simulink library "ddc_library"  (Simulink 6.2)
values from neighbouring files (symbols this model uses):
  num_fir_col = length(lpfir_coeff)/num_inputs    [ddc_mask.m]
libraries: xbsIndex_r3 x31, ddc_library x27, ddc_lo_lib x8
settings Model: LastModifiedBy=hchen05

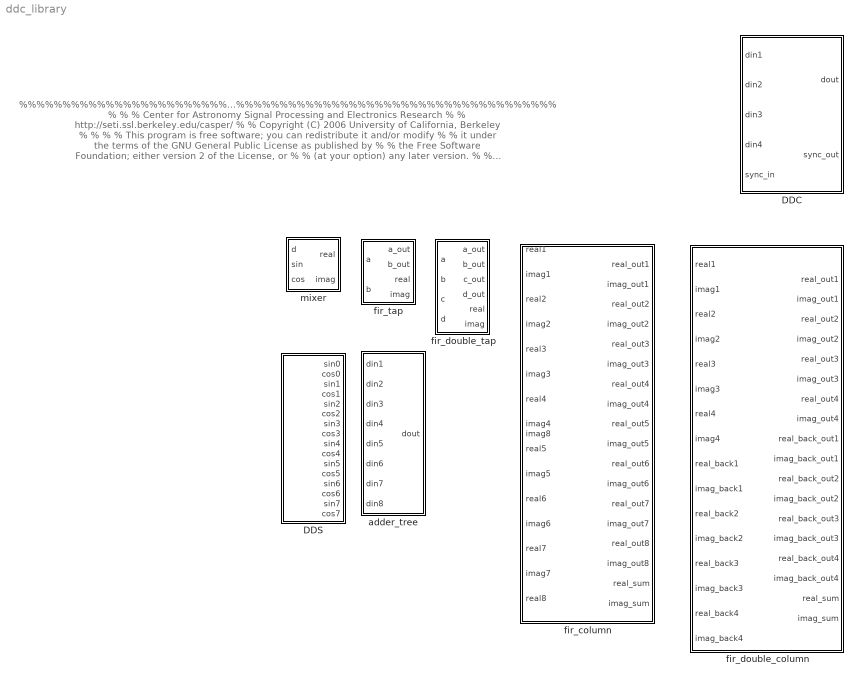
== system ddc_library ==
  note: %%%%%%%%%%%%%%%%%%%%%%%%%%%%%%%%%%%%%%%%%%%%%%%%%%%%%%%%%%%%%%%%%%%%%%%%%%%%%%%
      | %                                                                             %
      | %   Center for Astronomy Signal Processing and Electronics Research           %
      | %   http://seti.ssl.berkeley.edu/casper/                                      %
      | %   Copyright (C) 2006 University of California, Berkeley                     %
      | %                                                                             %
      | %   This program is free software; you can redistribute it and/or modify      %
      | %   it under the terms of the GNU General Public License as published by      %
      | %   the Free Software Foundation; either version 2 of the License, or         %
      | %   (at your option) any later version.                                       %
      | %                                                                             %
      | %   This program is distributed in the hope that it will be useful,           %
      | %   but WITHOUT ANY WARRANTY; without even the implied warranty of            %
      | %   MERCHANTABILITY or FITNESS FOR A PARTICULAR PURPOSE.  See the             %
      | %   GNU General Public License for more details.                              %
      | %                                                                             %
      | %   You should have received a copy of the GNU General Public License along   %
      | %   with this program; if not, write to the Free Software Foundation, Inc.,   %
      | %   51 Franklin Street, Fifth Floor, Boston, MA 02110-1301 USA.               %
      | %                                                                             %
      | %%%%%%%%%%%%%%%%%%%%%%%%%%%%%%%%%%%%%%%%%%%%%%%%%%%%%%%%%%%%%%%%%%%%%%%%%%%%%%%
  DDC : Subsystem  mask(DDC){freq_div=16, lo_freq=3, num_inputs=4, lo_bitwidth=18, lpfir_coeff=[1,zeros(1,15)], BitWidthOut=8, quantization=Round  (unbiased: +/- Inf), add_latency=2, mult_latency=3}
      mask prompts: freq_div "Frequency Divisions (M)"; lo_freq "LO Frequency (1/M*2pi)"; num_inputs "Inputs"; lo_bitwidth "LO BitWidth"; lpfir_coeff "FIR coefficients"; BitWidthOut "Bit Width Out"; quantization "Quantization Behavior"; add_latency "Add Latency"; mult_latency "Mult Latency"
      mask help: Decimating digital downconverter with parameterized LO and LPF coefficients.
      mask init:
      | ddc_mask;
      mask Help: eval('xlWeb([getenv(''MLIB_ROOT''), ''\astro_library\doc\ddc_usage.html''])')
      mask StyleString: edit,edit,edit,edit,edit,edit,popup(Truncate|Round  (unbiased: +/- Inf)|Round  (unbiased: Even Values)),edit,edit
  DDS : Subsystem  mask{freq_div=8, freq=2, num_lo=8, BitWidth=18, latency=2}
      mask prompts: freq_div "Frequency divisions (M)"; freq "Frequency (1/M*2pi)"; num_lo "Parallel LOs (N)"
      mask init:
      | dds_mask;
  adder_tree : Subsystem  mask{num_inputs=8, latency=2}
      mask prompts: num_inputs "Inputs"; latency "Latency per adder tree"
      mask init:
      | adder_tree_mask;
  fir_column : Subsystem  mask(fir_column){num_inputs=8, coeff=rand(128), mult_latency=2, add_latency=1}
      mask prompts: num_inputs "Inputs"; coeff "Coefficients"; mult_latency "Mult Latency"; add_latency "Add latency"
      mask init:
      | fir_column_mask;
  fir_double_column : Subsystem  mask(fir_double_column){num_inputs=4, coeff=rand(8), mult_latency=3, add_latency=2}
      mask prompts: num_inputs "Inputs"; coeff "Coefficients"; mult_latency "Mult Latency"; add_latency "Add latency"
      mask init:
      | fir_double_column_mask;
  fir_double_tap : Subsystem  mask(fir_double_tap){factor=0.073384, mult_latency=3, add_latency=2}
      mask prompts: mult_latency "Mult latency"; add_latency "Add latency"
  fir_tap : Subsystem  mask(fir_tap){factor=1, latency=3}
      mask prompts: latency "mult_latency"
  mixer : Subsystem  mask{BitWidth=18, latency=2}

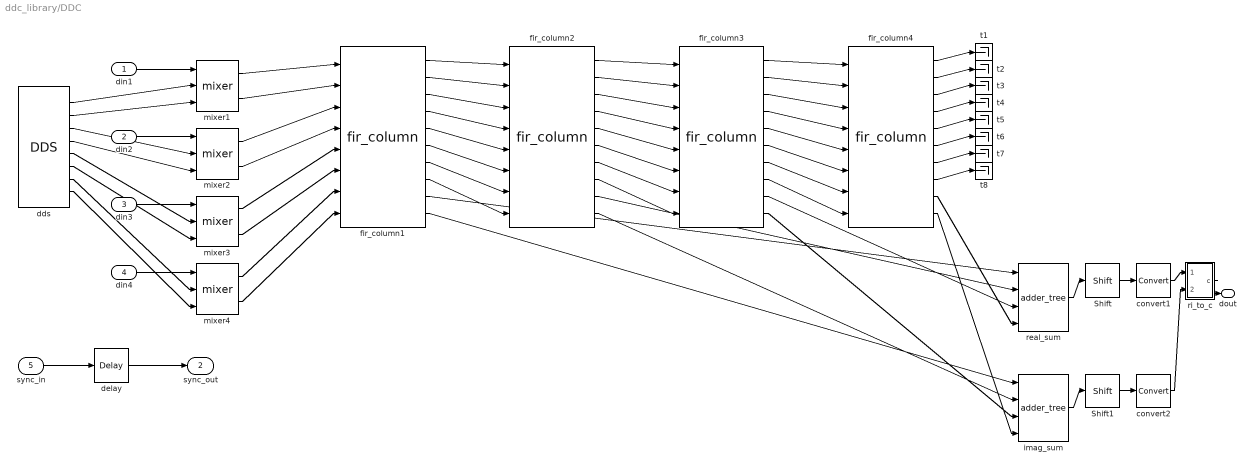
== system ddc_library/DDC ==
  din1 : Inport  Port=1  LatchInput=off
  din2 : Inport  Port=2  LatchInput=off
  din3 : Inport  Port=3  LatchInput=off
  din4 : Inport  Port=4  LatchInput=off
  sync_in : Inport  Port=5  LatchInput=off
  Shift : xbsIndex_r3/Shift  shift_dir=Left  shift_bits=1  precision=Full  arith_type="Signed  (2's comp)"  n_bits=8  bin_pt=2  quantization=Truncate  overflow=Wrap  latency=0  explicit_period=off  period=1  en=off  dbl_ovrd=off  show_param=off
      settings: xl_area=[0, 0, 0, 0, 0, 0, 0]
  Shift1 : xbsIndex_r3/Shift  shift_dir=Left  shift_bits=1  precision=Full  arith_type="Signed  (2's comp)"  n_bits=8  bin_pt=2  quantization=Truncate  overflow=Wrap  latency=0  explicit_period=off  period=1  en=off  dbl_ovrd=off  show_param=off
      settings: xl_area=[0, 0, 0, 0, 0, 0, 0]
  convert1 : xbsIndex_r3/Convert  arith_type="Signed  (2's comp)"  n_bits=BitWidthOut  bin_pt=BitWidthOut - 1  quantization="Round  (unbiased: +/- Inf)"  overflow=Saturate  latency=add_latency  explicit_period=on  period=1  dbl_ovrd=off  show_param=on  inserted_by_tool=off  pipeline=on
      settings: xl_area=[0, 0, 0, 0, 0, 0, 0]
  convert2 : xbsIndex_r3/Convert  arith_type="Signed  (2's comp)"  n_bits=BitWidthOut  bin_pt=BitWidthOut - 1  quantization="Round  (unbiased: +/- Inf)"  overflow=Saturate  latency=add_latency  explicit_period=on  period=1  dbl_ovrd=off  show_param=on  inserted_by_tool=off  pipeline=on
      settings: xl_area=[0, 0, 0, 0, 0, 0, 0]
  dds : ddc_library/DDS  freq_div=freq_div  freq=lo_freq  num_lo=num_inputs  BitWidth=lo_bitwidth  latency=2
      link override ddc_lo0/ddc_lo_const/const1: equ=P=C
  delay : xbsIndex_r3/Delay  latency=mult_latency*2+ceil(log2(num_inputs))*add_latency+ceil(log2(num_fir_col))*add_latency+add_latency  reg_retiming=off  explicit_period=off  period=1  en=off  accept_only_valid=off  init_zero=on  dbl_ovrd=off  show_param=off
      settings: xl_area=[0, 0, 0, 0, 0, 0, 0]
  fir_column1 : ddc_library/fir_column  num_inputs=num_inputs  coeff=lpfir_coeff(4:-1:1)  mult_latency=mult_latency  add_latency=1
  fir_column2 : ddc_library/fir_column  num_inputs=num_inputs  coeff=lpfir_coeff(8:-1:5)  mult_latency=mult_latency  add_latency=1
  fir_column3 : ddc_library/fir_column  num_inputs=num_inputs  coeff=lpfir_coeff(12:-1:9)  mult_latency=mult_latency  add_latency=1
  fir_column4 : ddc_library/fir_column  num_inputs=num_inputs  coeff=lpfir_coeff(16:-1:13)  mult_latency=mult_latency  add_latency=1
  imag_sum : ddc_library/adder_tree  num_inputs=4  latency=2
  mixer{1..4} (4 alike) : ddc_library/mixer  BitWidth=lo_bitwidth  latency=mult_latency
  real_sum : ddc_library/adder_tree  num_inputs=4  latency=2
  ri_to_c : Subsystem
  t{1..8} (8 alike) : Terminator
  dout : Outport
  sync_out : Outport  Port=2
  wires:
  real_sum/1 -> Shift/1
  imag_sum/1 -> Shift1/1
  Shift/1 -> convert1/1
  Shift1/1 -> convert2/1
  convert1/1 -> ri_to_c/1(re)
  convert2/1 -> ri_to_c/2(im)
  ri_to_c/1(c) -> dout/1
  sync_in/1 -> delay/1
  delay/1 -> sync_out/1
  din1/1 -> mixer1/1
  dds/1 -> mixer1/2
  dds/2 -> mixer1/3
  din2/1 -> mixer2/1
  dds/3 -> mixer2/2
  dds/4 -> mixer2/3
  din3/1 -> mixer3/1
  dds/5 -> mixer3/2
  dds/6 -> mixer3/3
  din4/1 -> mixer4/1
  dds/7 -> mixer4/2
  dds/8 -> mixer4/3
  mixer1/1 -> fir_column1/1
  mixer1/2 -> fir_column1/2
  mixer2/1 -> fir_column1/3
  mixer2/2 -> fir_column1/4
  mixer3/1 -> fir_column1/5
  mixer3/2 -> fir_column1/6
  mixer4/1 -> fir_column1/7
  mixer4/2 -> fir_column1/8
  fir_column1/9 -> real_sum/1
  fir_column1/10 -> imag_sum/1
  fir_column1/1 -> fir_column2/1
  fir_column1/2 -> fir_column2/2
  fir_column1/3 -> fir_column2/3
  fir_column1/4 -> fir_column2/4
  fir_column1/5 -> fir_column2/5
  fir_column1/6 -> fir_column2/6
  fir_column1/7 -> fir_column2/7
  fir_column1/8 -> fir_column2/8
  fir_column2/9 -> real_sum/2
  fir_column2/10 -> imag_sum/2
  fir_column2/1 -> fir_column3/1
  fir_column2/2 -> fir_column3/2
  fir_column2/3 -> fir_column3/3
  fir_column2/4 -> fir_column3/4
  fir_column2/5 -> fir_column3/5
  fir_column2/6 -> fir_column3/6
  fir_column2/7 -> fir_column3/7
  fir_column2/8 -> fir_column3/8
  fir_column3/9 -> real_sum/3
  fir_column3/10 -> imag_sum/3
  fir_column3/1 -> fir_column4/1
  fir_column3/2 -> fir_column4/2
  fir_column3/3 -> fir_column4/3
  fir_column3/4 -> fir_column4/4
  fir_column3/5 -> fir_column4/5
  fir_column3/6 -> fir_column4/6
  fir_column3/7 -> fir_column4/7
  fir_column3/8 -> fir_column4/8
  fir_column4/9 -> real_sum/4
  fir_column4/10 -> imag_sum/4
  fir_column4/1 -> t1/1
  fir_column4/2 -> t2/1
  fir_column4/3 -> t3/1
  fir_column4/4 -> t4/1
  fir_column4/5 -> t5/1
  fir_column4/6 -> t6/1
  fir_column4/7 -> t7/1
  fir_column4/8 -> t8/1

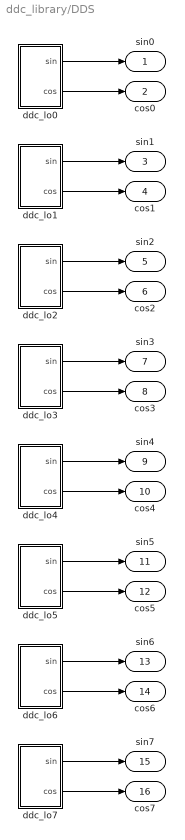
== system ddc_library/DDS ==
  ddc_lo0 : Subsystem  BlockChoice=ddc_lo_const
      link override ddc_lo_const: BitWidth=BitWidth  Phase=0
      link override ddc_lo_const/const1: equ=P=C
      link override ddc_lo_osc: BitWidth=BitWidth  counter_step=counter_step  counter_start=0  counter_width=counter_width  latency=latency
      settings: AttributesFormatString=%<BlockChoice>  TemplateBlock=ddc_lo_lib/ddc_lo  MemberBlocks=ddc_lo_const,ddc_lo_osc
  ddc_lo1 : Subsystem  BlockChoice=ddc_lo_const
      link override ddc_lo_const: BitWidth=BitWidth  Phase=1.5708
      link override ddc_lo_osc: BitWidth=BitWidth  counter_step=counter_step  counter_start=1  counter_width=counter_width  latency=latency
      settings: AttributesFormatString=%<BlockChoice>  TemplateBlock=ddc_lo_lib/ddc_lo  MemberBlocks=ddc_lo_const,ddc_lo_osc
  ddc_lo2 : Subsystem  BlockChoice=ddc_lo_const
      link override ddc_lo_const: BitWidth=BitWidth  Phase=3.1416
      link override ddc_lo_osc: BitWidth=BitWidth  counter_step=counter_step  counter_start=2  counter_width=counter_width  latency=latency
      settings: AttributesFormatString=%<BlockChoice>  TemplateBlock=ddc_lo_lib/ddc_lo  MemberBlocks=ddc_lo_const,ddc_lo_osc
  ddc_lo3 : Subsystem  BlockChoice=ddc_lo_const
      link override ddc_lo_const: BitWidth=BitWidth  Phase=4.7124
      link override ddc_lo_osc: BitWidth=BitWidth  counter_step=counter_step  counter_start=3  counter_width=counter_width  latency=latency
      settings: AttributesFormatString=%<BlockChoice>  TemplateBlock=ddc_lo_lib/ddc_lo  MemberBlocks=ddc_lo_const,ddc_lo_osc
  ddc_lo4 : Subsystem  BlockChoice=ddc_lo_const
      link override ddc_lo_const: BitWidth=BitWidth  Phase=6.2832
      settings: AttributesFormatString=%<BlockChoice>  TemplateBlock=ddc_lo_lib/ddc_lo  MemberBlocks=ddc_lo_const,ddc_lo_osc
  ddc_lo5 : Subsystem  BlockChoice=ddc_lo_const
      link override ddc_lo_const: BitWidth=BitWidth  Phase=7.854
      settings: AttributesFormatString=%<BlockChoice>  TemplateBlock=ddc_lo_lib/ddc_lo  MemberBlocks=ddc_lo_const,ddc_lo_osc
  ddc_lo6 : Subsystem  BlockChoice=ddc_lo_const
      link override ddc_lo_const: BitWidth=BitWidth  Phase=9.4248
      settings: AttributesFormatString=%<BlockChoice>  TemplateBlock=ddc_lo_lib/ddc_lo  MemberBlocks=ddc_lo_const,ddc_lo_osc
  ddc_lo7 : Subsystem  BlockChoice=ddc_lo_const
      link override ddc_lo_const: BitWidth=BitWidth  Phase=10.9956
      settings: AttributesFormatString=%<BlockChoice>  TemplateBlock=ddc_lo_lib/ddc_lo  MemberBlocks=ddc_lo_const,ddc_lo_osc
  sin0 : Outport
  cos0 : Outport  Port=2
  sin1 : Outport  Port=3
  cos1 : Outport  Port=4
  sin2 : Outport  Port=5
  cos2 : Outport  Port=6
  sin3 : Outport  Port=7
  cos3 : Outport  Port=8
  sin4 : Outport  Port=9
  cos4 : Outport  Port=10
  sin5 : Outport  Port=11
  cos5 : Outport  Port=12
  sin6 : Outport  Port=13
  cos6 : Outport  Port=14
  sin7 : Outport  Port=15
  cos7 : Outport  Port=16
  wires:
  ddc_lo0/1(sin) -> sin0/1
  ddc_lo0/2(cos) -> cos0/1
  ddc_lo1/1(sin) -> sin1/1
  ddc_lo1/2(cos) -> cos1/1
  ddc_lo2/1(sin) -> sin2/1
  ddc_lo2/2(cos) -> cos2/1
  ddc_lo3/1(sin) -> sin3/1
  ddc_lo3/2(cos) -> cos3/1
  ddc_lo4/1(sin) -> sin4/1
  ddc_lo4/2(cos) -> cos4/1
  ddc_lo5/1(sin) -> sin5/1
  ddc_lo5/2(cos) -> cos5/1
  ddc_lo6/1(sin) -> sin6/1
  ddc_lo6/2(cos) -> cos6/1
  ddc_lo7/1(sin) -> sin7/1
  ddc_lo7/2(cos) -> cos7/1

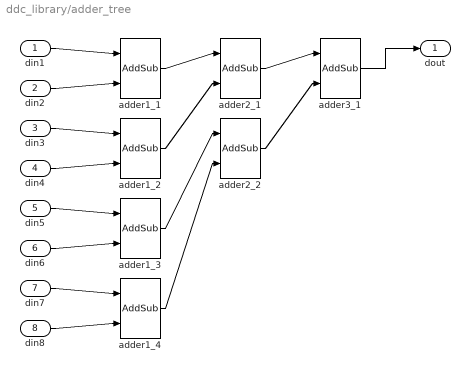
== system ddc_library/adder_tree ==
  din1 : Inport  Port=1  LatchInput=off
  din2 : Inport  Port=2  LatchInput=off
  din3 : Inport  Port=3  LatchInput=off
  din4 : Inport  Port=4  LatchInput=off
  din5 : Inport  Port=5  LatchInput=off
  din6 : Inport  Port=6  LatchInput=off
  din7 : Inport  Port=7  LatchInput=off
  din8 : Inport  Port=8  LatchInput=off
  adder1_{1..4} (4 alike) : xbsIndex_r3/AddSub  mode=Addition  precision=Full  arith_type=Unsigned  n_bits=8  bin_pt=2  quantization=Truncate  overflow=Wrap  latency=latency  explicit_period=off  period=1  use_carryin=off  use_carryout=off  en=off  dbl_ovrd=off  show_param=off  use_core=on  pipeline=on  use_rpm=on  gen_core=off
      settings: xl_area=[0, 0, 0, 0, 0, 0, 0]
  adder2_1 : xbsIndex_r3/AddSub  mode=Addition  precision=Full  arith_type=Unsigned  n_bits=8  bin_pt=2  quantization=Truncate  overflow=Wrap  latency=latency  explicit_period=off  period=1  use_carryin=off  use_carryout=off  en=off  dbl_ovrd=off  show_param=off  use_core=on  pipeline=on  use_rpm=on  gen_core=off
      settings: xl_area=[0, 0, 0, 0, 0, 0, 0]
  adder2_2 : xbsIndex_r3/AddSub  mode=Addition  precision=Full  arith_type=Unsigned  n_bits=8  bin_pt=2  quantization=Truncate  overflow=Wrap  latency=latency  explicit_period=off  period=1  use_carryin=off  use_carryout=off  en=off  dbl_ovrd=off  show_param=off  use_core=on  pipeline=on  use_rpm=on  gen_core=off
      settings: xl_area=[0, 0, 0, 0, 0, 0, 0]
  adder3_1 : xbsIndex_r3/AddSub  mode=Addition  precision=Full  arith_type=Unsigned  n_bits=8  bin_pt=2  quantization=Truncate  overflow=Wrap  latency=latency  explicit_period=off  period=1  use_carryin=off  use_carryout=off  en=off  dbl_ovrd=off  show_param=off  use_core=on  pipeline=on  use_rpm=on  gen_core=off
      settings: xl_area=[0, 0, 0, 0, 0, 0, 0]
  dout : Outport
  wires:
  din1/1 -> adder1_1/1
  din2/1 -> adder1_1/2
  din3/1 -> adder1_2/1
  din4/1 -> adder1_2/2
  din5/1 -> adder1_3/1
  din6/1 -> adder1_3/2
  din7/1 -> adder1_4/1
  din8/1 -> adder1_4/2
  adder1_1/1 -> adder2_1/1
  adder1_2/1 -> adder2_1/2
  adder1_3/1 -> adder2_2/1
  adder1_4/1 -> adder2_2/2
  adder2_1/1 -> adder3_1/1
  adder2_2/1 -> adder3_1/2
  adder3_1/1 -> dout/1

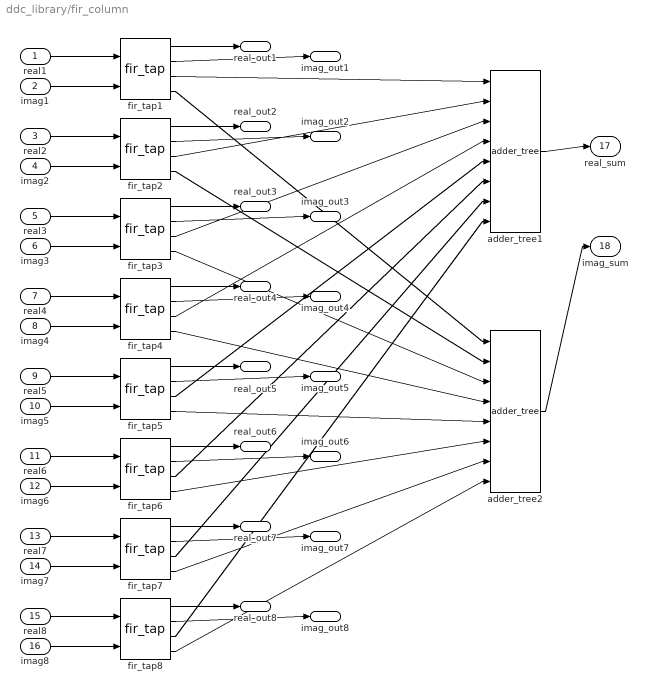
== system ddc_library/fir_column ==
  real1 : Inport  Port=1  LatchInput=off
  imag1 : Inport  Port=2  LatchInput=off
  real2 : Inport  Port=3  LatchInput=off
  imag2 : Inport  Port=4  LatchInput=off
  real3 : Inport  Port=5  LatchInput=off
  imag3 : Inport  Port=6  LatchInput=off
  real4 : Inport  Port=7  LatchInput=off
  imag4 : Inport  Port=8  LatchInput=off
  real5 : Inport  Port=9  LatchInput=off
  imag5 : Inport  Port=10  LatchInput=off
  real6 : Inport  Port=11  LatchInput=off
  imag6 : Inport  Port=12  LatchInput=off
  real7 : Inport  Port=13  LatchInput=off
  imag7 : Inport  Port=14  LatchInput=off
  real8 : Inport  Port=15  LatchInput=off
  imag8 : Inport  Port=16  LatchInput=off
  adder_tree1 : ddc_library/adder_tree  num_inputs=num_inputs  latency=add_latency
  adder_tree2 : ddc_library/adder_tree  num_inputs=num_inputs  latency=add_latency
  fir_tap1 : ddc_library/fir_tap  factor=coeff(1)  latency=mult_latency
  fir_tap2 : ddc_library/fir_tap  factor=coeff(2)  latency=mult_latency
  fir_tap3 : ddc_library/fir_tap  factor=coeff(3)  latency=mult_latency
  fir_tap4 : ddc_library/fir_tap  factor=coeff(4)  latency=mult_latency
  fir_tap5 : ddc_library/fir_tap  factor=coeff(5)  latency=mult_latency
  fir_tap6 : ddc_library/fir_tap  factor=coeff(6)  latency=mult_latency
  fir_tap7 : ddc_library/fir_tap  factor=coeff(7)  latency=mult_latency
  fir_tap8 : ddc_library/fir_tap  factor=coeff(8)  latency=mult_latency
  real_out1 : Outport
  imag_out1 : Outport  Port=2
  real_out2 : Outport  Port=3
  imag_out2 : Outport  Port=4
  real_out3 : Outport  Port=5
  imag_out3 : Outport  Port=6
  real_out4 : Outport  Port=7
  imag_out4 : Outport  Port=8
  real_out5 : Outport  Port=9
  imag_out5 : Outport  Port=10
  real_out6 : Outport  Port=11
  imag_out6 : Outport  Port=12
  real_out7 : Outport  Port=13
  imag_out7 : Outport  Port=14
  real_out8 : Outport  Port=15
  imag_out8 : Outport  Port=16
  real_sum : Outport  Port=17
  imag_sum : Outport  Port=18
  wires:
  adder_tree1/1 -> real_sum/1
  adder_tree2/1 -> imag_sum/1
  real1/1 -> fir_tap1/1
  imag1/1 -> fir_tap1/2
  fir_tap1/1 -> real_out1/1
  fir_tap1/2 -> imag_out1/1
  fir_tap1/3 -> adder_tree1/1
  fir_tap1/4 -> adder_tree2/1
  real2/1 -> fir_tap2/1
  imag2/1 -> fir_tap2/2
  fir_tap2/1 -> real_out2/1
  fir_tap2/2 -> imag_out2/1
  fir_tap2/3 -> adder_tree1/2
  fir_tap2/4 -> adder_tree2/2
  real3/1 -> fir_tap3/1
  imag3/1 -> fir_tap3/2
  fir_tap3/1 -> real_out3/1
  fir_tap3/2 -> imag_out3/1
  fir_tap3/3 -> adder_tree1/3
  fir_tap3/4 -> adder_tree2/3
  real4/1 -> fir_tap4/1
  imag4/1 -> fir_tap4/2
  fir_tap4/1 -> real_out4/1
  fir_tap4/2 -> imag_out4/1
  fir_tap4/3 -> adder_tree1/4
  fir_tap4/4 -> adder_tree2/4
  real5/1 -> fir_tap5/1
  imag5/1 -> fir_tap5/2
  fir_tap5/1 -> real_out5/1
  fir_tap5/2 -> imag_out5/1
  fir_tap5/3 -> adder_tree1/5
  fir_tap5/4 -> adder_tree2/5
  real6/1 -> fir_tap6/1
  imag6/1 -> fir_tap6/2
  fir_tap6/1 -> real_out6/1
  fir_tap6/2 -> imag_out6/1
  fir_tap6/3 -> adder_tree1/6
  fir_tap6/4 -> adder_tree2/6
  real7/1 -> fir_tap7/1
  imag7/1 -> fir_tap7/2
  fir_tap7/1 -> real_out7/1
  fir_tap7/2 -> imag_out7/1
  fir_tap7/3 -> adder_tree1/7
  fir_tap7/4 -> adder_tree2/7
  real8/1 -> fir_tap8/1
  imag8/1 -> fir_tap8/2
  fir_tap8/1 -> real_out8/1
  fir_tap8/2 -> imag_out8/1
  fir_tap8/3 -> adder_tree1/8
  fir_tap8/4 -> adder_tree2/8

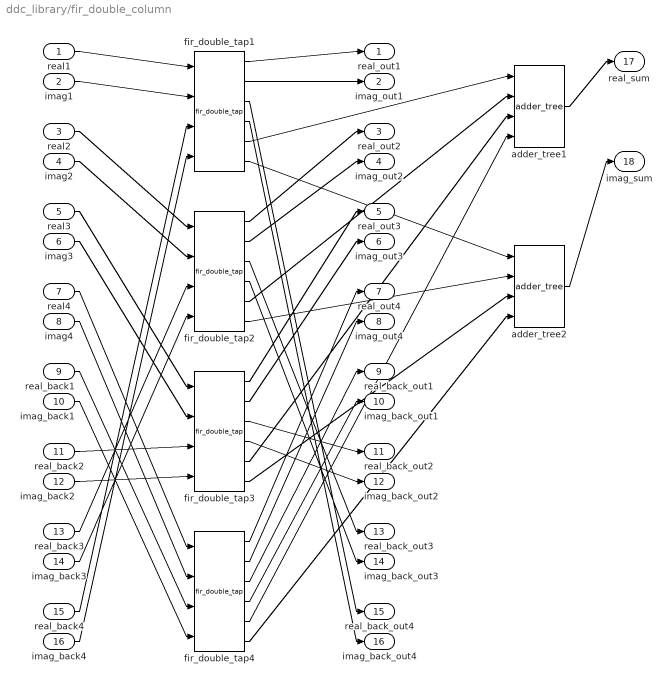
== system ddc_library/fir_double_column ==
  real1 : Inport  Port=1  LatchInput=off
  imag1 : Inport  Port=2  LatchInput=off
  real2 : Inport  Port=3  LatchInput=off
  imag2 : Inport  Port=4  LatchInput=off
  real3 : Inport  Port=5  LatchInput=off
  imag3 : Inport  Port=6  LatchInput=off
  real4 : Inport  Port=7  LatchInput=off
  imag4 : Inport  Port=8  LatchInput=off
  real_back1 : Inport  Port=9  LatchInput=off
  imag_back1 : Inport  Port=10  LatchInput=off
  real_back2 : Inport  Port=11  LatchInput=off
  imag_back2 : Inport  Port=12  LatchInput=off
  real_back3 : Inport  Port=13  LatchInput=off
  imag_back3 : Inport  Port=14  LatchInput=off
  real_back4 : Inport  Port=15  LatchInput=off
  imag_back4 : Inport  Port=16  LatchInput=off
  adder_tree1 : ddc_library/adder_tree  num_inputs=num_inputs  latency=add_latency
  adder_tree2 : ddc_library/adder_tree  num_inputs=num_inputs  latency=add_latency
  fir_double_tap1 : ddc_library/fir_double_tap  factor=coeff(1)  mult_latency=mult_latency  add_latency=add_latency
  fir_double_tap2 : ddc_library/fir_double_tap  factor=coeff(2)  mult_latency=mult_latency  add_latency=add_latency
  fir_double_tap3 : ddc_library/fir_double_tap  factor=coeff(3)  mult_latency=mult_latency  add_latency=add_latency
  fir_double_tap4 : ddc_library/fir_double_tap  factor=coeff(4)  mult_latency=mult_latency  add_latency=add_latency
  real_out1 : Outport
  imag_out1 : Outport  Port=2
  real_out2 : Outport  Port=3
  imag_out2 : Outport  Port=4
  real_out3 : Outport  Port=5
  imag_out3 : Outport  Port=6
  real_out4 : Outport  Port=7
  imag_out4 : Outport  Port=8
  real_back_out1 : Outport  Port=9
  imag_back_out1 : Outport  Port=10
  real_back_out2 : Outport  Port=11
  imag_back_out2 : Outport  Port=12
  real_back_out3 : Outport  Port=13
  imag_back_out3 : Outport  Port=14
  real_back_out4 : Outport  Port=15
  imag_back_out4 : Outport  Port=16
  real_sum : Outport  Port=17
  imag_sum : Outport  Port=18
  wires:
  adder_tree1/1 -> real_sum/1
  adder_tree2/1 -> imag_sum/1
  real1/1 -> fir_double_tap1/1
  imag1/1 -> fir_double_tap1/2
  real_back4/1 -> fir_double_tap1/3
  imag_back4/1 -> fir_double_tap1/4
  fir_double_tap1/1 -> real_out1/1
  fir_double_tap1/2 -> imag_out1/1
  fir_double_tap1/3 -> real_back_out4/1
  fir_double_tap1/4 -> imag_back_out4/1
  fir_double_tap1/5 -> adder_tree1/1
  fir_double_tap1/6 -> adder_tree2/1
  real2/1 -> fir_double_tap2/1
  imag2/1 -> fir_double_tap2/2
  real_back3/1 -> fir_double_tap2/3
  imag_back3/1 -> fir_double_tap2/4
  fir_double_tap2/1 -> real_out2/1
  fir_double_tap2/2 -> imag_out2/1
  fir_double_tap2/3 -> real_back_out3/1
  fir_double_tap2/4 -> imag_back_out3/1
  fir_double_tap2/5 -> adder_tree1/2
  fir_double_tap2/6 -> adder_tree2/2
  real3/1 -> fir_double_tap3/1
  imag3/1 -> fir_double_tap3/2
  real_back2/1 -> fir_double_tap3/3
  imag_back2/1 -> fir_double_tap3/4
  fir_double_tap3/1 -> real_out3/1
  fir_double_tap3/2 -> imag_out3/1
  fir_double_tap3/3 -> real_back_out2/1
  fir_double_tap3/4 -> imag_back_out2/1
  fir_double_tap3/5 -> adder_tree1/3
  fir_double_tap3/6 -> adder_tree2/3
  real4/1 -> fir_double_tap4/1
  imag4/1 -> fir_double_tap4/2
  real_back1/1 -> fir_double_tap4/3
  imag_back1/1 -> fir_double_tap4/4
  fir_double_tap4/1 -> real_out4/1
  fir_double_tap4/2 -> imag_out4/1
  fir_double_tap4/3 -> real_back_out1/1
  fir_double_tap4/4 -> imag_back_out1/1
  fir_double_tap4/5 -> adder_tree1/4
  fir_double_tap4/6 -> adder_tree2/4

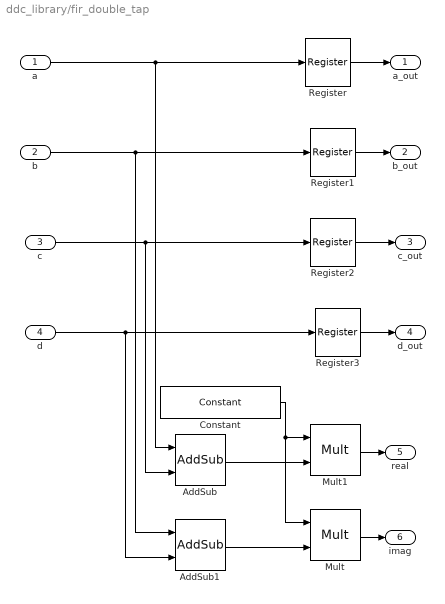
== system ddc_library/fir_double_tap ==
  a : Inport  Port=1  LatchInput=off
  b : Inport  Port=2  LatchInput=off
  c : Inport  Port=3  LatchInput=off
  d : Inport  Port=4  LatchInput=off
  AddSub : xbsIndex_r3/AddSub  mode=Addition  precision=User Defined  arith_type="Signed  (2's comp)"  n_bits=18  bin_pt=16  quantization=Truncate  overflow=Wrap  latency=add_latency  explicit_period=on  period=1  use_carryin=off  use_carryout=off  en=off  dbl_ovrd=off  show_param=off  use_core=on  pipeline=off  use_rpm=on  gen_core=off
      settings: xl_area=[0, 0, 0, 0, 0, 0, 0]
  AddSub1 : xbsIndex_r3/AddSub  mode=Addition  precision=User Defined  arith_type="Signed  (2's comp)"  n_bits=18  bin_pt=16  quantization=Truncate  overflow=Wrap  latency=add_latency  explicit_period=on  period=1  use_carryin=off  use_carryout=off  en=off  dbl_ovrd=off  show_param=off  use_core=on  pipeline=off  use_rpm=on  gen_core=off
      settings: xl_area=[0, 0, 0, 0, 0, 0, 0]
  Constant : xbsIndex_r3/Constant  const=factor  equ=P=C  arith_type="Signed  (2's comp)"  n_bits=18  bin_pt=17  opselect=C  inp2=PCIN>>17  opr=+  inp1=P  carry=CIN  iostate=0  explicit_period=on  period=1  dbl_ovrd=off
  Mult : xbsIndex_r3/Mult  precision=Full  arith_type="Signed  (2's comp)"  n_bits=18  bin_pt=17  quantization=Truncate  overflow=Wrap  latency=mult_latency  explicit_period=off  period=1  en=off  dbl_ovrd=off  show_param=on  mult_type=Parallel  oversample=2  use_embedded=on  pipeline=on  use_rpm=off  placement_style=Rectangular Shape  gen_core=off
      settings: xl_area=[0, 0, 0, 0, 0, 0, 0]
  Mult1 : xbsIndex_r3/Mult  precision=Full  arith_type="Signed  (2's comp)"  n_bits=18  bin_pt=17  quantization=Truncate  overflow=Wrap  latency=mult_latency  explicit_period=off  period=1  en=off  dbl_ovrd=off  show_param=on  mult_type=Parallel  oversample=2  use_embedded=on  pipeline=on  use_rpm=off  placement_style=Rectangular Shape  gen_core=off
      settings: xl_area=[0, 0, 0, 0, 0, 0, 0]
  Register{,1..3} (4 alike) : xbsIndex_r3/Register  init=0  reg_only_valid=off  explicit_period=on  period=1  rst=off  en=off  out_en=off  dbl_ovrd=off  show_param=off
      settings: xl_area=[0, 0, 0, 0, 0, 0, 0]
  a_out : Outport
  b_out : Outport  Port=2
  c_out : Outport  Port=3
  d_out : Outport  Port=4
  real : Outport  Port=5
  imag : Outport  Port=6
  wires:
  Register1/1 -> b_out/1
  Register/1 -> a_out/1
  Constant/1 -> Mult/1, Mult1/1
  Mult/1 -> imag/1
  Mult1/1 -> real/1
  Register3/1 -> d_out/1
  Register2/1 -> c_out/1
  a/1 -> Register/1, AddSub/1
  b/1 -> Register1/1, AddSub1/1
  c/1 -> Register2/1, AddSub/2
  d/1 -> Register3/1, AddSub1/2
  AddSub/1 -> Mult1/2
  AddSub1/1 -> Mult/2

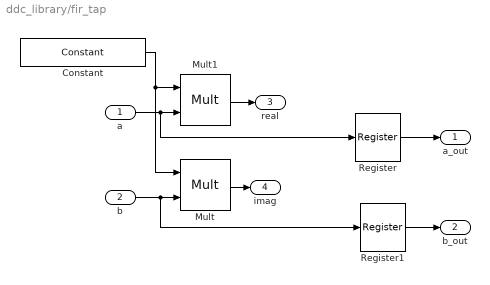
== system ddc_library/fir_tap ==
  a : Inport  Port=1  LatchInput=off
  b : Inport  Port=2  LatchInput=off
  Constant : xbsIndex_r3/Constant  const=factor  equ=P=C  arith_type="Signed  (2's comp)"  n_bits=18  bin_pt=17  opselect=C  inp2=PCIN>>17  opr=+  inp1=P  carry=CIN  iostate=0  explicit_period=on  period=1  dbl_ovrd=off
  Mult : xbsIndex_r3/Mult  precision=Full  arith_type="Signed  (2's comp)"  n_bits=18  bin_pt=17  quantization=Truncate  overflow=Wrap  latency=latency  explicit_period=on  period=1  en=off  dbl_ovrd=off  show_param=on  mult_type=Parallel  oversample=2  use_embedded=on  pipeline=on  use_rpm=off  placement_style=Rectangular Shape  gen_core=off
      settings: xl_area=[0, 0, 0, 0, 0, 0, 0]
  Mult1 : xbsIndex_r3/Mult  precision=Full  arith_type="Signed  (2's comp)"  n_bits=18  bin_pt=17  quantization=Truncate  overflow=Wrap  latency=latency  explicit_period=on  period=1  en=off  dbl_ovrd=off  show_param=on  mult_type=Parallel  oversample=2  use_embedded=on  pipeline=on  use_rpm=off  placement_style=Rectangular Shape  gen_core=off
      settings: xl_area=[0, 0, 0, 0, 0, 0, 0]
  Register : xbsIndex_r3/Register  init=0  reg_only_valid=off  explicit_period=on  period=1  rst=off  en=off  out_en=off  dbl_ovrd=off  show_param=off
      settings: xl_area=[0, 0, 0, 0, 0, 0, 0]
  Register1 : xbsIndex_r3/Register  init=0  reg_only_valid=off  explicit_period=on  period=1  rst=off  en=off  out_en=off  dbl_ovrd=off  show_param=off
      settings: xl_area=[0, 0, 0, 0, 0, 0, 0]
  a_out : Outport
  b_out : Outport  Port=2
  real : Outport  Port=3
  imag : Outport  Port=4
  wires:
  Mult1/1 -> real/1
  b/1 -> Mult/2, Register1/1
  Mult/1 -> imag/1
  a/1 -> Mult1/2, Register/1
  Constant/1 -> Mult1/1, Mult/1
  Register/1 -> a_out/1
  Register1/1 -> b_out/1

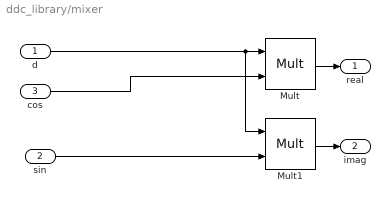
== system ddc_library/mixer ==
  d : Inport  Port=1  LatchInput=off
  sin : Inport  Port=2  LatchInput=off
  cos : Inport  Port=3  LatchInput=off
  Mult : xbsIndex_r3/Mult  precision=Full  arith_type="Signed  (2's comp)"  n_bits=BitWidth  bin_pt=BitWidth-1  quantization=Truncate  overflow=Wrap  latency=latency  explicit_period=off  period=1  en=off  dbl_ovrd=off  show_param=on  mult_type=Parallel  oversample=2  use_embedded=on  pipeline=on  use_rpm=off  placement_style=Rectangular Shape  gen_core=off
      settings: xl_area=[0, 0, 0, 0, 0, 0, 0]
  Mult1 : xbsIndex_r3/Mult  precision=Full  arith_type="Signed  (2's comp)"  n_bits=BitWidth  bin_pt=BitWidth-1  quantization=Truncate  overflow=Wrap  latency=latency  explicit_period=off  period=1  en=off  dbl_ovrd=off  show_param=on  mult_type=Parallel  oversample=2  use_embedded=on  pipeline=on  use_rpm=off  placement_style=Rectangular Shape  gen_core=off
      settings: xl_area=[0, 0, 0, 0, 0, 0, 0]
  real : Outport
  imag : Outport  Port=2
  wires:
  d/1 -> Mult/1, Mult1/1
  Mult/1 -> real/1
  cos/1 -> Mult/2
  Mult1/1 -> imag/1
  sin/1 -> Mult1/2

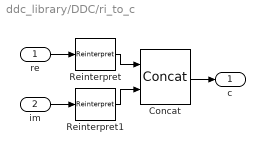
== system ddc_library/DDC/ri_to_c ==
  re : Inport  Port=1  LatchInput=off
  im : Inport  Port=2  LatchInput=off
  Concat : xbsIndex_r3/Concat  num_inputs=2  explicit_period=off  period=1  dbl_ovrd=off
  Reinterpret : xbsIndex_r3/Reinterpret  force_arith_type=on  arith_type=Unsigned  force_bin_pt=on  bin_pt=0  force_valid=on
  Reinterpret1 : xbsIndex_r3/Reinterpret  force_arith_type=on  arith_type=Unsigned  force_bin_pt=on  bin_pt=0  force_valid=on
  c : Outport
  wires:
  im/1 -> Reinterpret1/1
  Concat/1 -> c/1
  re/1 -> Reinterpret/1
  Reinterpret1/1 -> Concat/2
  Reinterpret/1 -> Concat/1

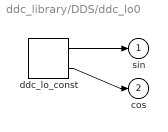
== system ddc_library/DDS/ddc_lo0 ==
  ddc_lo_const : ddc_lo_lib/ddc_lo_const  BitWidth=BitWidth  Phase=0
  sin : Outport
  cos : Outport  Port=2
  wires:
  ddc_lo_const/1 -> sin/1
  ddc_lo_const/2 -> cos/1

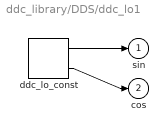
== system ddc_library/DDS/ddc_lo1 ==
  ddc_lo_const : ddc_lo_lib/ddc_lo_const  BitWidth=BitWidth  Phase=1.5708
  sin : Outport
  cos : Outport  Port=2
  wires:
  ddc_lo_const/1 -> sin/1
  ddc_lo_const/2 -> cos/1

== system ddc_library/DDS/ddc_lo2 ==
  ddc_lo_const : ddc_lo_lib/ddc_lo_const  BitWidth=BitWidth  Phase=3.1416
  sin : Outport
  cos : Outport  Port=2
  wires:
  ddc_lo_const/1 -> sin/1
  ddc_lo_const/2 -> cos/1

== system ddc_library/DDS/ddc_lo3 ==
  ddc_lo_const : ddc_lo_lib/ddc_lo_const  BitWidth=BitWidth  Phase=4.7124
  sin : Outport
  cos : Outport  Port=2
  wires:
  ddc_lo_const/1 -> sin/1
  ddc_lo_const/2 -> cos/1

== system ddc_library/DDS/ddc_lo4 ==
  ddc_lo_const : ddc_lo_lib/ddc_lo_const  BitWidth=BitWidth  Phase=6.2832
  sin : Outport
  cos : Outport  Port=2
  wires:
  ddc_lo_const/1 -> sin/1
  ddc_lo_const/2 -> cos/1

== system ddc_library/DDS/ddc_lo5 ==
  ddc_lo_const : ddc_lo_lib/ddc_lo_const  BitWidth=BitWidth  Phase=7.854
  sin : Outport
  cos : Outport  Port=2
  wires:
  ddc_lo_const/1 -> sin/1
  ddc_lo_const/2 -> cos/1

== system ddc_library/DDS/ddc_lo6 ==
  ddc_lo_const : ddc_lo_lib/ddc_lo_const  BitWidth=BitWidth  Phase=9.4248
  sin : Outport
  cos : Outport  Port=2
  wires:
  ddc_lo_const/1 -> sin/1
  ddc_lo_const/2 -> cos/1

== system ddc_library/DDS/ddc_lo7 ==
  ddc_lo_const : ddc_lo_lib/ddc_lo_const  BitWidth=BitWidth  Phase=10.9956
  sin : Outport
  cos : Outport  Port=2
  wires:
  ddc_lo_const/1 -> sin/1
  ddc_lo_const/2 -> cos/1
